simulink model "InverseKinematicsRREstimation"  (R2022b)
settings: Solver=ode23  StartTime=0.0  StopTime=10  RelTol=1e-7  AbsTol=1e-7
settings Model: Creator=aless  LastModifiedBy=aless

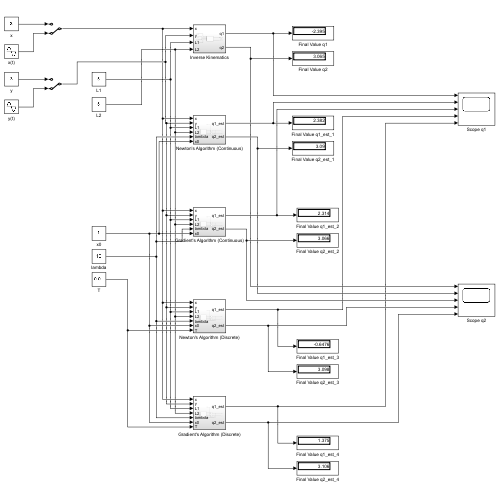
[thumbnail: Simulink's stored preview of the top-level diagram]
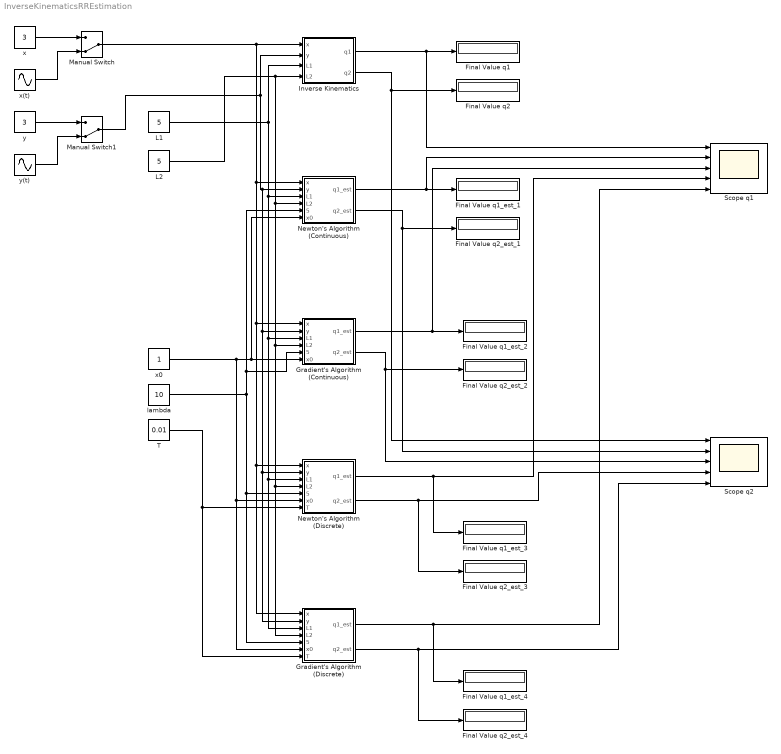
== system InverseKinematicsRREstimation ==
  Final Value q1 : Display
  Final Value q1_est_{1..4} (4 alike) : Display
  Final Value q2 : Display
  Final Value q2_est_{1..4} (4 alike) : Display
  Gradient's Algorithm (Continuous) : Subsystem
  Gradient's Algorithm (Discrete) : Subsystem
  Inverse Kinematics : Subsystem
  L1 : Constant  Value=5
  L2 : Constant  Value=5
  Manual Switch : ManualSwitch  CurrentSetting=0
  Manual Switch1 : ManualSwitch  CurrentSetting=0
  Newton's Algorithm (Continuous) : Subsystem
  Newton's Algorithm (Discrete) : Subsystem
  Scope q1 : Scope  NumInputPorts=5
  Scope q2 : Scope  NumInputPorts=5
  T : Constant  Value=0.01
  lambda : Constant  Value=10
  x : Constant  Value=3
  x(t) : Sin  Amplitude=0.5  SampleTime=0
  x0 : Constant
  y : Constant  Value=3
  y(t) : Sin  Amplitude=0.5  SampleTime=0
  wires:
  Manual Switch/1 -> Gradient's Algorithm (Discrete)/1(x), Newton's Algorithm (Discrete)/1(x), Gradient's Algorithm (Continuous)/1(x), Newton's Algorithm (Continuous)/1(x), Inverse Kinematics/1(x)
  lambda/1 -> Newton's Algorithm (Continuous)/5(lambda), Gradient's Algorithm (Continuous)/5(lambda), Gradient's Algorithm (Discrete)/5(lambda), Newton's Algorithm (Discrete)/5(lambda)
  Newton's Algorithm (Continuous)/1(q1_est) -> Final Value q1_est_1/1, Scope q1/2
  Inverse Kinematics/1(q1) -> Scope q1/1, Final Value q1/1
  x0/1 -> Gradient's Algorithm (Discrete)/6(x0), Newton's Algorithm (Discrete)/6(x0), Newton's Algorithm (Continuous)/6(x0), Gradient's Algorithm (Continuous)/6(x0)
  Inverse Kinematics/2(q2) -> Scope q2/1, Final Value q2/1
  Manual Switch1/1 -> Inverse Kinematics/2(y), Newton's Algorithm (Continuous)/2(y), Gradient's Algorithm (Discrete)/2(y), Newton's Algorithm (Discrete)/2(y), Gradient's Algorithm (Continuous)/2(y)
  L1/1 -> Inverse Kinematics/3(L1), Gradient's Algorithm (Discrete)/3(L1), Newton's Algorithm (Discrete)/3(L1), Gradient's Algorithm (Continuous)/3(L1), Newton's Algorithm (Continuous)/3(L1)
  L2/1 -> Gradient's Algorithm (Discrete)/4(L2), Newton's Algorithm (Discrete)/4(L2), Gradient's Algorithm (Continuous)/4(L2), Newton's Algorithm (Continuous)/4(L2), Inverse Kinematics/4(L2)
  Newton's Algorithm (Continuous)/2(q2_est) -> Scope q2/2, Final Value q2_est_1/1
  Gradient's Algorithm (Continuous)/1(q1_est) -> Scope q1/3, Final Value q1_est_2/1
  Gradient's Algorithm (Continuous)/2(q2_est) -> Scope q2/3, Final Value q2_est_2/1
  T/1 -> Gradient's Algorithm (Discrete)/7(T), Newton's Algorithm (Discrete)/7(T)
  Newton's Algorithm (Discrete)/2(q2_est) -> Scope q2/4, Final Value q2_est_3/1
  Newton's Algorithm (Discrete)/1(q1_est) -> Scope q1/4, Final Value q1_est_3/1
  Gradient's Algorithm (Discrete)/2(q2_est) -> Scope q2/5, Final Value q2_est_4/1
  Gradient's Algorithm (Discrete)/1(q1_est) -> Scope q1/5, Final Value q1_est_4/1
  x/1 -> Manual Switch/1
  x(t)/1 -> Manual Switch/2
  y/1 -> Manual Switch1/1
  y(t)/1 -> Manual Switch1/2

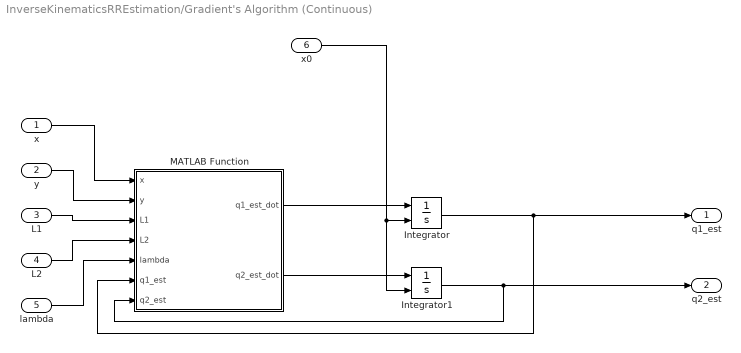
== system InverseKinematicsRREstimation/Gradient's Algorithm (Continuous) ==
  x : Inport
  y : Inport  Port=2
  L1 : Inport  Port=3
  L2 : Inport  Port=4
  lambda : Inport  Port=5
  x0 : Inport  Port=6
  Integrator : Integrator  InitialConditionSource=external  InitialCondition=0.1
  Integrator1 : Integrator  InitialConditionSource=external  InitialCondition=0.1
  MATLAB Function : MATLAB Function  TreatAsAtomicUnit=on
  q1_est : Outport
  q2_est : Outport  Port=2
  wires:
  x/1 -> MATLAB Function/1(x)
  lambda/1 -> MATLAB Function/5(lambda)
  MATLAB Function/1(q1_est_dot) -> Integrator/1
  Integrator/1 -> MATLAB Function/6(q1_est), q1_est/1
  x0/1 -> Integrator1/2, Integrator/2
  MATLAB Function/2(q2_est_dot) -> Integrator1/1
  Integrator1/1 -> MATLAB Function/7(q2_est), q2_est/1
  L1/1 -> MATLAB Function/3(L1)
  y/1 -> MATLAB Function/2(y)
  L2/1 -> MATLAB Function/4(L2)

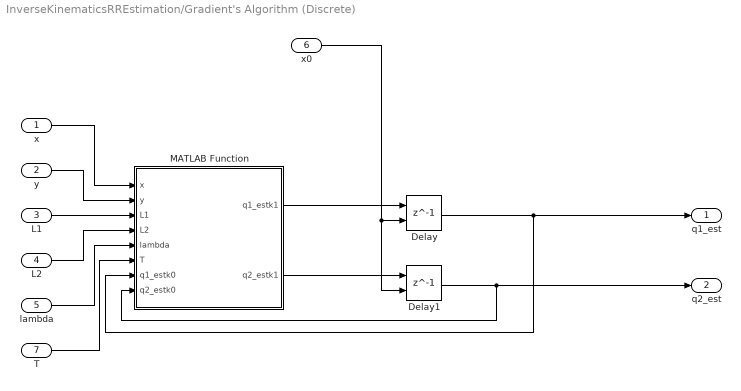
== system InverseKinematicsRREstimation/Gradient's Algorithm (Discrete) ==
  x : Inport
  y : Inport  Port=2
  L1 : Inport  Port=3
  L2 : Inport  Port=4
  lambda : Inport  Port=5
  x0 : Inport  Port=6
  T : Inport  Port=7
  Delay : Delay  DelayLength=1  InitialConditionSource=Input port  SampleTime=0.1
      settings: InputPortMap=u0,p4
  Delay1 : Delay  DelayLength=1  InitialConditionSource=Input port  SampleTime=0.1
      settings: InputPortMap=u0,p4
  MATLAB Function : MATLAB Function  TreatAsAtomicUnit=on
  q1_est : Outport
  q2_est : Outport  Port=2
  wires:
  x/1 -> MATLAB Function/1(x)
  lambda/1 -> MATLAB Function/5(lambda)
  MATLAB Function/1(q1_estk1) -> Delay/1
  Delay/1 -> MATLAB Function/7(q1_estk0), q1_est/1
  x0/1 -> Delay1/2, Delay/2
  L1/1 -> MATLAB Function/3(L1)
  y/1 -> MATLAB Function/2(y)
  L2/1 -> MATLAB Function/4(L2)
  T/1 -> MATLAB Function/6(T)
  MATLAB Function/2(q2_estk1) -> Delay1/1
  Delay1/1 -> MATLAB Function/8(q2_estk0), q2_est/1

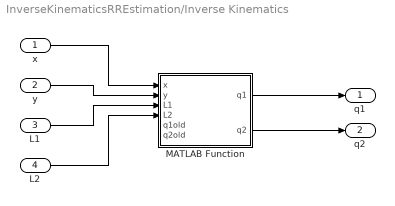
== system InverseKinematicsRREstimation/Inverse Kinematics ==
  x : Inport
  y : Inport  Port=2
  L1 : Inport  Port=3
  L2 : Inport  Port=4
  MATLAB Function : MATLAB Function  TreatAsAtomicUnit=on
  q1 : Outport
  q2 : Outport  Port=2
  wires:
  x/1 -> MATLAB Function/1(x)
  MATLAB Function/1(q1) -> q1/1
  y/1 -> MATLAB Function/2(y)
  L1/1 -> MATLAB Function/3(L1)
  L2/1 -> MATLAB Function/4(L2)
  MATLAB Function/2(q2) -> q2/1

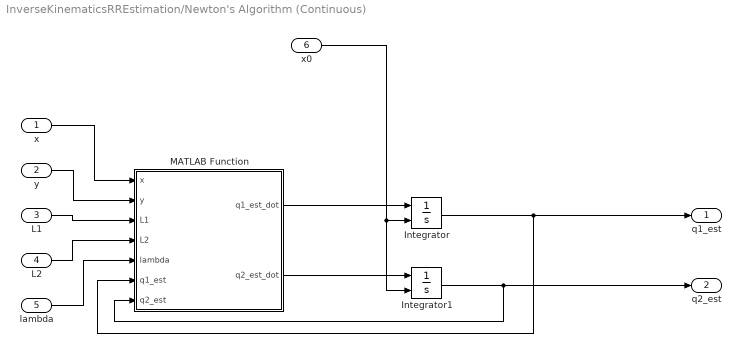
== system InverseKinematicsRREstimation/Newton's Algorithm (Continuous) ==
  x : Inport
  y : Inport  Port=2
  L1 : Inport  Port=3
  L2 : Inport  Port=4
  lambda : Inport  Port=5
  x0 : Inport  Port=6
  Integrator : Integrator  InitialConditionSource=external  InitialCondition=0.1
  Integrator1 : Integrator  InitialConditionSource=external  InitialCondition=0.1
  MATLAB Function : MATLAB Function  TreatAsAtomicUnit=on
  q1_est : Outport
  q2_est : Outport  Port=2
  wires:
  x/1 -> MATLAB Function/1(x)
  lambda/1 -> MATLAB Function/5(lambda)
  MATLAB Function/1(q1_est_dot) -> Integrator/1
  Integrator/1 -> MATLAB Function/6(q1_est), q1_est/1
  x0/1 -> Integrator1/2, Integrator/2
  MATLAB Function/2(q2_est_dot) -> Integrator1/1
  Integrator1/1 -> MATLAB Function/7(q2_est), q2_est/1
  L1/1 -> MATLAB Function/3(L1)
  y/1 -> MATLAB Function/2(y)
  L2/1 -> MATLAB Function/4(L2)

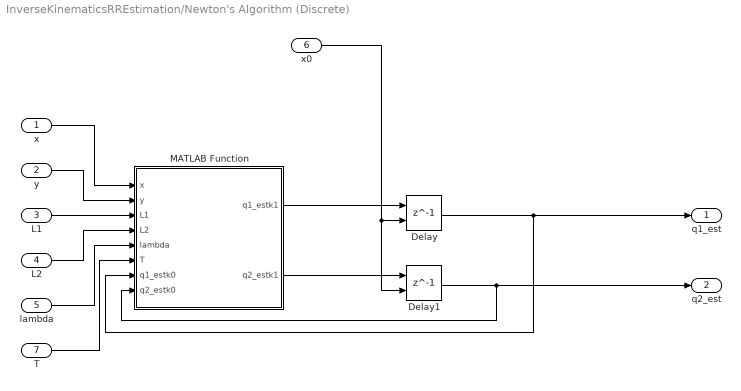
== system InverseKinematicsRREstimation/Newton's Algorithm (Discrete) ==
  x : Inport
  y : Inport  Port=2
  L1 : Inport  Port=3
  L2 : Inport  Port=4
  lambda : Inport  Port=5
  x0 : Inport  Port=6
  T : Inport  Port=7
  Delay : Delay  DelayLength=1  InitialConditionSource=Input port  SampleTime=0.1
      settings: InputPortMap=u0,p4
  Delay1 : Delay  DelayLength=1  InitialConditionSource=Input port  SampleTime=0.1
      settings: InputPortMap=u0,p4
  MATLAB Function : MATLAB Function  TreatAsAtomicUnit=on
  q1_est : Outport
  q2_est : Outport  Port=2
  wires:
  x/1 -> MATLAB Function/1(x)
  lambda/1 -> MATLAB Function/5(lambda)
  MATLAB Function/1(q1_estk1) -> Delay/1
  Delay/1 -> MATLAB Function/7(q1_estk0), q1_est/1
  x0/1 -> Delay1/2, Delay/2
  L1/1 -> MATLAB Function/3(L1)
  y/1 -> MATLAB Function/2(y)
  L2/1 -> MATLAB Function/4(L2)
  T/1 -> MATLAB Function/6(T)
  MATLAB Function/2(q2_estk1) -> Delay1/1
  Delay1/1 -> MATLAB Function/8(q2_estk0), q2_est/1

== matlab function InverseKinematicsRREstimation/Newton's Algorithm (Discrete)/MATLAB Function ==
  data: x input; y input; L1 input; L2 input; q1_estk1 output; lambda input; T input; q1_estk0 input; q2_estk0 input; q2_estk1 output
function [q1_estk1, q2_estk1] = fcn(x, y, L1, L2, lambda, T, q1_estk0, q2_estk0)
jacobian = [-L2*sin(q1_estk0+q2_estk0)-L1*sin(q1_estk0), -L2*sin(q1_estk0+q2_estk0);
            +L2*cos(q1_estk0+q2_estk0)+L1*cos(q1_estk0), +L2*cos(q1_estk0+q2_estk0)];

Hq_est = [L2*cos(q1_estk0+q2_estk0)+L1*cos(q1_estk0);
          L2*sin(q1_estk0+q2_estk0)+L1*sin(q1_estk0)];

q_est_k1 = [q1_estk0; q2_estk0] + T*(lambda/2 * inv(jacobian) * ([x; y] - Hq_est));

q1_estk1 = q_est_k1(1);
q2_estk1 = q_est_k1(2);

== matlab function InverseKinematicsRREstimation/Newton's Algorithm (Continuous)/MATLAB Function ==
  data: x input; y input; L1 input; L2 input; q1_est_dot output; lambda input; q1_est input; q2_est input; q2_est_dot output
function [q1_est_dot, q2_est_dot] = fcn(x, y, L1, L2, lambda, q1_est, q2_est)
jacobian = [-L2*sin(q1_est+q2_est)-L1*sin(q1_est), -L2*sin(q1_est+q2_est);
            +L2*cos(q1_est+q2_est)+L1*cos(q1_est), +L2*cos(q1_est+q2_est)];

Hq_est = [L2*cos(q1_est+q2_est)+L1*cos(q1_est);
     L2*sin(q1_est+q2_est)+L1*sin(q1_est)];

q_est_dot = lambda/2 * inv(jacobian) * ([x; y] - Hq_est);

q1_est_dot = q_est_dot(1);
q2_est_dot = q_est_dot(2);

== matlab function InverseKinematicsRREstimation/Gradient's Algorithm (Discrete)/MATLAB Function ==
  data: x input; y input; L1 input; L2 input; q1_estk1 output; lambda input; T input; q1_estk0 input; q2_estk0 input; q2_estk1 output
function [q1_estk1, q2_estk1] = fcn(x, y, L1, L2, lambda, T, q1_estk0, q2_estk0)
jacobian = [-L2*sin(q1_estk0+q2_estk0)-L1*sin(q1_estk0), -L2*sin(q1_estk0+q2_estk0);
            +L2*cos(q1_estk0+q2_estk0)+L1*cos(q1_estk0), +L2*cos(q1_estk0+q2_estk0)];

Hq_est = [L2*cos(q1_estk0+q2_estk0)+L1*cos(q1_estk0);
          L2*sin(q1_estk0+q2_estk0)+L1*sin(q1_estk0)];

q_est_k1 = [q1_estk0; q2_estk0] + T*(lambda/2 * (jacobian)' * ([x; y] - Hq_est));

q1_estk1 = q_est_k1(1);
q2_estk1 = q_est_k1(2);

== matlab function InverseKinematicsRREstimation/Inverse Kinematics/MATLAB Function ==
  data: x input; q1 output; y input; L1 input; L2 input; q2 output; q1old input; q2old input
function [q1, q2] = fcn(x, y, L1, L2, q1old, q2old)

a = (x^2 + y^2 - L1^2 - L2^2)/(2*L1*L2);
q2 = atan2(+sqrt(1 - a^2), a);

c = cos(q2)*L2 + L1;
d = sin(q2)*L2;

q1 = atan2(c*y - d*x, c*x + d*y);

== matlab function InverseKinematicsRREstimation/Gradient's Algorithm (Continuous)/MATLAB Function ==
  data: x input; y input; L1 input; L2 input; q1_est_dot output; lambda input; q1_est input; q2_est input; q2_est_dot output
function [q1_est_dot, q2_est_dot] = fcn(x, y, L1, L2, lambda, q1_est, q2_est)
jacobian = [-L2*sin(q1_est+q2_est)-L1*sin(q1_est), -L2*sin(q1_est+q2_est);
            +L2*cos(q1_est+q2_est)+L1*cos(q1_est), +L2*cos(q1_est+q2_est)];

Hq_est = [L2*cos(q1_est+q2_est)+L1*cos(q1_est);
     L2*sin(q1_est+q2_est)+L1*sin(q1_est)];

q_est_dot = lambda/2 * (jacobian)' * ([x; y] - Hq_est);

q1_est_dot = q_est_dot(1);
q2_est_dot = q_est_dot(2);
